simulink model "controladorRampa"  (R2024b)
settings: Solver=VariableStepAuto  StartTime=0.0  StopTime=50  RelTol=1e-3
values from neighbouring files (symbols this model uses):
  planta = obterPlanta()    [obterMalhaAngular.m]    (also in obterMalhaTangencial.m; simularBarra.m)
  saturacoes = obterSaturacao()    [simularBarra.m]
  x0 = tr_req    [ajustarRequisitosEstabilidade.m]
undefined symbols (not defined in the file or in its folder): controlador, theta0
libraries: slpidlib x1
settings Model: Creator=josal  LastModifiedBy=josal

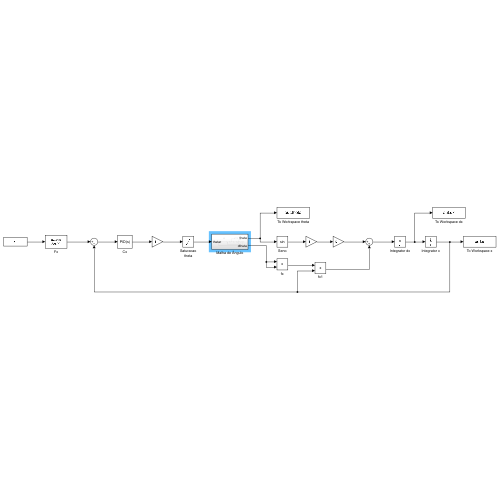
[thumbnail: Simulink's stored preview of the top-level diagram]
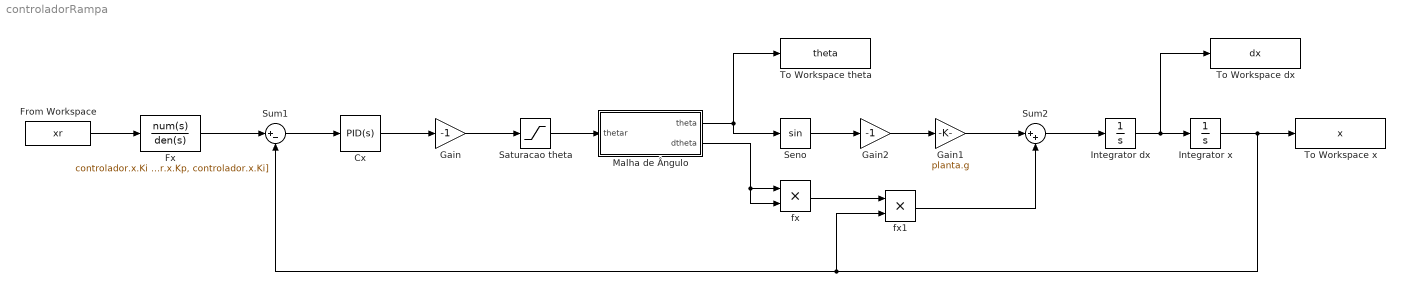
== system controladorRampa ==
  Cx : slpidlib/PID Controller  Controller=PID  Form=Parallel  TimeDomain=Continuous-time  UseExternalTs=off  SampleTime=-1  IntegratorMethod=Forward Euler  FilterMethod=Forward Euler  ControllerParametersSource=internal  P=controlador.x.Kp  I=controlador.x.Ki  UseKiTs=off  D=controlador.x.Kd  UseExternalDerivativeSource=off  N=100  UseFilter=on  TunerSelectOption=Transfer Function Based (PID Tuner App)  InitialConditionSource=internal  InitialConditionForIntegrator=0  InitialConditionForFilter=0  DifferentiatorICPrevScaledInput=0  ExternalReset=none  TrackingMode=off  Kt=1  LimitOutput=off  SatLimitsSource=internal  UpperSaturationLimit=saturacoes.sat_theta  LowerSaturationLimit=-saturacoes.sat_theta  LinearizeAsGain=on  AntiWindupMode=back-calculation  Kb=10  LimitIntegrator=off  UpperIntegratorSaturationLimit=inf  LowerIntegratorSaturationLimit=-inf  POutMin=[]  POutMax=[]  IOutMin=[]  IOutMax=[]  DOutMin=[]  DOutMax=[]  NOutMin=[]  NOutMax=[]  SumOutMin=[]  SumOutMax=[]  SaturationOutMin=[]  SaturationOutMax=[]  PParamMin=[]  PParamMax=[]  IParamMin=[]  IParamMax=[]  DParamMin=[]  DParamMax=[]  NParamMin=[]  NParamMax=[]  KbParamMin=[]  KbParamMax=[]  KtParamMin=[]  KtParamMax=[]  KbOutMin=[]  KbOutMax=[]  KtOutMin=[]  KtOutMax=[]  IntegratorOutMin=[]  IntegratorOutMax=[]  FilterOutMin=[]  FilterOutMax=[]  SumI1OutMin=[]  SumI1OutMax=[]  SumI2OutMin=[]  SumI2OutMax=[]  SumI3OutMin=[]  SumI3OutMax=[]  SumI4OutMin=[]  SumI4OutMax=[]  SumDOutMin=[]  SumDOutMax=[]  DifferentiatorOutMin=[]  DifferentiatorOutMax=[]  FilterDiffOutCoefMin=[]  FilterDiffOutCoefMax=[]  ReciprocalOutMin=[]  ReciprocalOutMax=[]  SumDenOutMin=[]  SumDenOutMax=[]  SumNumOutMin=[]  SumNumOutMax=[]  DivideOutMin=[]  DivideOutMax=[]  UdiffTsProdOutMin=[]  UdiffTsProdOutMax=[]  NTsProdOutMin=[]  NTsProdOutMax=[]  UintegralTsProdOutMin=[]  UintegralTsProdOutMax=[]  UngainTsProdOutMin=[]  UngainTsProdOutMax=[]  ClampingZeroOutDataTypeStr=Inherit: Inherit via back propagation  ClampingZeroOutMin=[]  ClampingZeroOutMax=[]  FilterDenConstantOutDataTypeStr=Inherit: Inherit via back propagation  FilterDenConstantOutMin=[]  FilterDenConstantOutMax=[]  PCopyOutDataTypeStr=Inherit: Inherit via back propagation  PCopyOutMin=[]  PCopyOutMax=[]  NCopyOutDataTypeStr=Inherit: Inherit via back propagation  NCopyOutMin=[]  NCopyOutMax=[]  IntegratorContinuousStateAttributes=''  IntegratorStateMustResolveToSignalObject=off  IntegratorRTWStateStorageClass=Auto  FilterContinuousStateAttributes=''  FilterStateMustResolveToSignalObject=off  FilterRTWStateStorageClass=Auto  ParallelPVariant=InternalParameters  IdealPVariant=Disabled  IVariant=InternalParameters  DVariant=InternalParameters  IntegratorVariant=Continuous  SatVariant=Disabled  AWVariant=Passthrough  PCopyVariant=Disabled  TRVariant=Disabled  FdbkBlocksVariant=Forward  IdealPFdbkVariant=Disabled  SatFdbkVariant=Disabled  DerivativeFilterVariant=ContFilter  NVariant=InternalParameters  NCopyVariant=Disabled  FilterICVariant=InternalICsFilter  IntegratorICVariant=InternalICs  ExternalResetVariant=Disabled  TRSumVariant=Passthrough  SumFdbkVariant=Disabled  SumVariant=Sum_PID  TsampFilterVariant=InternalTs  TsampNgainVariant=Passthrough  TsampIntegralVariant=Disabled_SignalSpec  ExternalSaturationOutDataTypeStr=Inherit: Same as second input  DerivativeSourceVariant=ErrorSignal  PreIntVariant=InternalPreInt
  From Workspace : FromWorkspace  VariableName=xr
  Fx : TransferFcn  Numerator=controlador.x.Ki  Denominator=[controlador.x.Kd, controlador.x.Kp, controlador.x.Ki]
  Gain : Gain  Gain=-1
  Gain1 : Gain  Gain=planta.g
  Gain2 : Gain  Gain=-1
  Integrator dx : Integrator
  Integrator x : Integrator  InitialCondition=x0
  Malha de Ângulo : Subsystem
  Saturacao theta : Saturate  UpperLimit=saturacoes.sat_theta  LowerLimit=-saturacoes.sat_theta
  Seno : Trigonometry
  Sum1 : Sum  Inputs=|+-
  Sum2 : Sum  Inputs=|++
  To Workspace dx : ToWorkspace  VariableName=dx  SaveFormat=Structure With Time  SampleTime=-1
  To Workspace theta : ToWorkspace  VariableName=theta  SaveFormat=Structure With Time  SampleTime=-1
  To Workspace x : ToWorkspace  VariableName=x  SaveFormat=Structure With Time  SampleTime=-1
  fx : Product
  fx1 : Product
  wires:
  From Workspace/1 -> Fx/1
  Fx/1 -> Sum1/1
  Sum1/1 -> Cx/1
  Integrator dx/1 -> To Workspace dx/1, Integrator x/1
  Integrator x/1 -> To Workspace x/1, fx1/2, Sum1/2
  Cx/1 -> Gain/1
  Malha de Ângulo/1(theta) -> Seno/1, To Workspace theta/1
  Seno/1 -> Gain2/1
  Gain2/1 -> Gain1/1
  Malha de Ângulo/2(dtheta) -> fx/2, fx/1
  fx/1 -> fx1/1
  Gain1/1 -> Sum2/1
  Sum2/1 -> Integrator dx/1
  Gain/1 -> Saturacao theta/1
  Saturacao theta/1 -> Malha de Ângulo/1(thetar)
  fx1/1 -> Sum2/2

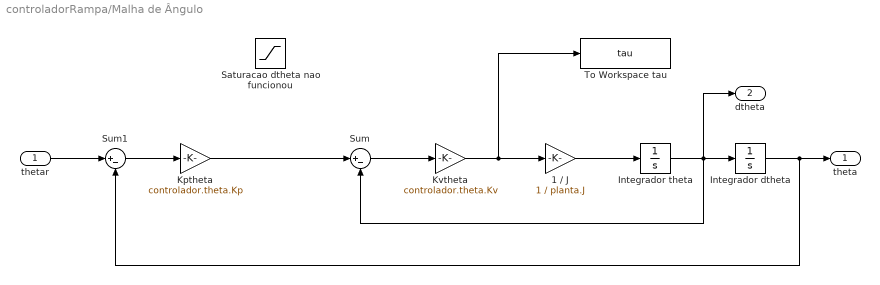
== system controladorRampa/Malha de Ângulo ==
  thetar : Inport
  1 / J : Gain  Gain=1 / planta.J
  Integrador dtheta : Integrator
  Integrador theta : Integrator  InitialCondition=theta0
  Kptheta : Gain  Gain=controlador.theta.Kp
  Kvtheta : Gain  Gain=controlador.theta.Kv
  Saturacao dtheta nao funcionou : Saturate  UpperLimit=saturacoes.sat_dtheta  LowerLimit=-saturacoes.sat_dtheta
  Sum : Sum  Inputs=|+-
  Sum1 : Sum  Inputs=|+-
  To Workspace tau : ToWorkspace  VariableName=tau  SaveFormat=Structure With Time  SampleTime=-1
  theta : Outport
  dtheta : Outport  Port=2
  wires:
  Integrador theta/1 -> dtheta/1, Sum/2, Integrador dtheta/1
  Sum1/1 -> Kptheta/1
  Integrador dtheta/1 -> Sum1/2, theta/1
  Kvtheta/1 -> 1 / J/1, To Workspace tau/1
  thetar/1 -> Sum1/1
  1 / J/1 -> Integrador theta/1
  Sum/1 -> Kvtheta/1
  Kptheta/1 -> Sum/1
